simulink model "aggregated_junctions"  (R2020a)
settings: Solver=FixedStepDiscrete  StartTime=0.0  StopTime=0.2  FixedStep=0.1  RelTol=1e-3  EnableMultiTasking=on
settings Model: Creator=BEAR  LastModifiedBy=bzhan
settings SolverCC: AutoInsertRateTranBlk=on
settings DataIOCC: LimitDataPoints=on  ReturnWorkspaceOutputs=off
settings OptimizationCC: LifeSpan=inf
settings DebuggingCC: AllowSymbolicDim=off  SFUnexpectedBacktrackingDiag=warning  SFNoUnconditionalDefaultTransitionDiag=warning  SFExecutionAtInitializationDiag=none  ArithmeticOperatorsInVariantConditions=warning
settings SFSimCC: SimUseLocalCustomCode=off  CustomCodeUndefinedFunction=UseInterfaceOnly
settings RTWCC: RTWUseLocalCustomCode=off
settings CodeAppCC: StateflowObjectComments=on
settings GRTTargetCC: TargetLangStandard=C89/C90 (ANSI)
settings ConfigComp: CovMetricSettings=dw  CovHtmlReporting=on  CovSaveCumulativeToWorkspaceVar=on  CovSaveSingleToWorkspaceVar=on  CovShowResultsExplorer=off  CovExternalEMLEnable=off  CovSFcnEnable=off

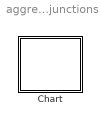
== system aggregated_junctions ==
  Chart : Stateflow chart  TreatAsAtomicUnit=on

== stateflow chart aggregated_junctions/Chart ==
  state A
    en: f("enA")
    ex: f("exA")
  state C
  state B
    en: f("enB")
    ex: f("exB")
  (default) -> A : {x=1}
  A -> (junction 5) [order 1] : [x==0]{f("conAJun")}/{f("tranAJun")}
  A -> B [order 2]
  (junction 5) -> C : {f("conJunC")}/{f("tranJunC")}
  B -> (junction 5) : {f("conBJun")}/{f("tranBJun")}
  data: s function_input; x local
  function f(s):
    | function f(s)
    |     fprintf(s+"\n");
